simulink model "hf_point_mass_subsonic_airplane"  (R2024b)
settings: Solver=ode45  StartTime=0.0  StopTime=5*60  RelTol=1e-3  AbsTol=1e-6
values from neighbouring files (symbols this model uses):
  FPS2MPH = 3600/5280    (= 0.681818181818)    [luckep2.m]
  RAD2DEG = 180/pi    (= 57.2957795131)    [luckep2.m]
undefined symbols (not defined in the file or in its folder): gd, ic, params
libraries: simulink_extras x5, dspstat3 x1, simulink x1
(part 1 of 2)
settings Model: Creator=jdlarson1  LastModifiedBy=Benjamin Lucke
settings SolverCC: AlgebraicLoopSolver=TrustRegion
settings DataIOCC: SaveFormat=Array  SignalLoggingSaveFormat=ModelDataLogs  ReturnWorkspaceOutputs=off
settings OptimizationCC: BlockReduction=off  BooleanDataType=off  ReuseModelBlockBuffer=off
settings DebuggingCC: SaveWithParameterizedLinksMsg=none  UnderspecifiedInitializationDetection=Classic  MergeDetectMultiDrivingBlocksExec=none  SignalResolutionControl=TryResolveAllWithWarning  MultiTaskDSMMsg=warning  MultiTaskCondExecSysMsg=none  UnconnectedInputMsg=warning  UnconnectedOutputMsg=warning  UnconnectedLineMsg=warning
settings HardwareCC: TargetUnknown=on
settings ModelReferenceCC: EnableRefExpFcnMdlSchedulingChecks=on  PropagateSignalLabelsOutOfModel=off
settings RTWCC: GPUComputeCapability=3.5  DLArmComputeVersion=19.05
settings GRTTargetCC: CombineOutputUpdateFcns=off  GRTInterface=on

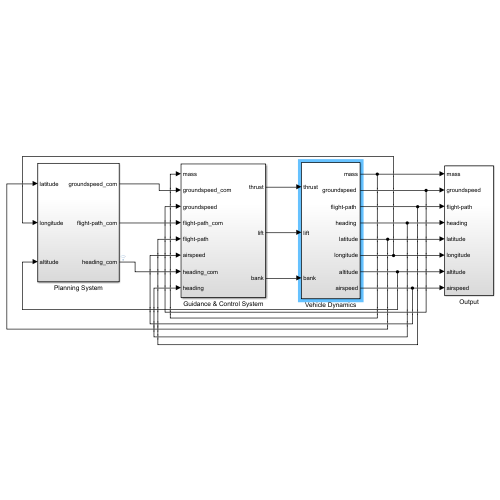
[thumbnail: Simulink's stored preview of the top-level diagram]
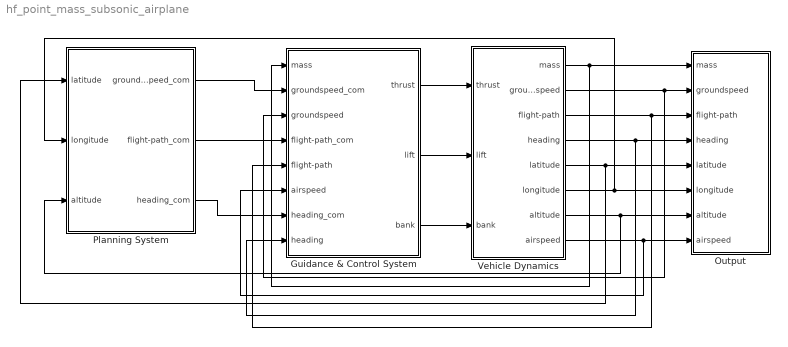
== system hf_point_mass_subsonic_airplane ==
  Guidance & Control System : Subsystem
  Output : Subsystem
  Planning System : Subsystem
  Vehicle Dynamics : Subsystem
  wires:
  Guidance & Control System/3(bank) -> Vehicle Dynamics/3(bank)
  Vehicle Dynamics/1(" mass") -> Output/1(mass), Guidance & Control System/1(mass)
  Guidance & Control System/2(lift) -> Vehicle Dynamics/2("lift ")
  Guidance & Control System/1(thrust) -> Vehicle Dynamics/1("thrust ")
  Planning System/1(groundspeed_com) -> Guidance & Control System/2(groundspeed_com)
  Planning System/2(flight-path_com) -> Guidance & Control System/4(flight-path_com)
  Planning System/3(heading_com) -> Guidance & Control System/7(heading_com)
  Vehicle Dynamics/4(" heading ") -> Guidance & Control System/8(heading), Output/4(heading)
  Vehicle Dynamics/3(" flight-path ") -> Guidance & Control System/5(flight-path), Output/3(flight-path)
  Vehicle Dynamics/2(" groundspeed ") -> Guidance & Control System/3(groundspeed), Output/2(groundspeed)
  Vehicle Dynamics/8(airspeed) -> Guidance & Control System/6(airspeed), Output/8(airspeed)
  Vehicle Dynamics/7(altitude) -> Planning System/3(altitude), Output/7(altitude)
  Vehicle Dynamics/6(longitude) -> Planning System/2(longitude), Output/6(longitude)
  Vehicle Dynamics/5(latitude) -> Planning System/1(latitude), Output/5(latitude)

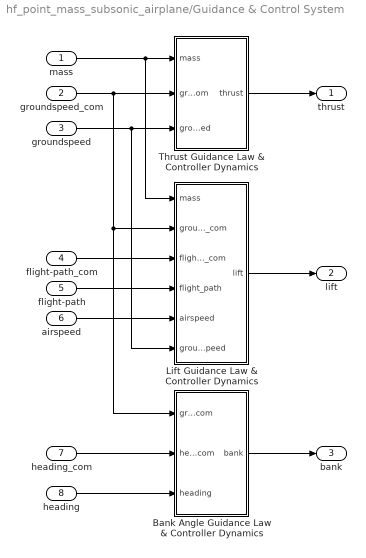
== system hf_point_mass_subsonic_airplane/Guidance & Control System ==
  mass : Inport
  groundspeed_com : Inport  Port=2
  groundspeed : Inport  Port=3
  flight-path_com : Inport  Port=4
  flight-path : Inport  Port=5
  airspeed : Inport  Port=6
  heading_com : Inport  Port=7
  heading : Inport  Port=8
  Bank Angle Guidance Law & Controller Dynamics : Subsystem
  Lift Guidance Law & Controller Dynamics : Subsystem
  Thrust Guidance Law & Controller Dynamics : Subsystem
  thrust : Outport
  lift : Outport  Port=2
  bank : Outport  Port=3
  wires:
  mass/1 -> Lift Guidance Law & Controller Dynamics/1(mass), Thrust Guidance Law & Controller Dynamics/1(mass)
  heading_com/1 -> Bank Angle Guidance Law & Controller Dynamics/2(heading_com)
  groundspeed/1 -> Thrust Guidance Law & Controller Dynamics/3(groundspeed), Lift Guidance Law & Controller Dynamics/6(groundspeed)
  groundspeed_com/1 -> Lift Guidance Law & Controller Dynamics/2(groundspeed_com), Bank Angle Guidance Law & Controller Dynamics/1(groundspeed_com), Thrust Guidance Law & Controller Dynamics/2(groundspeed_com)
  heading/1 -> Bank Angle Guidance Law & Controller Dynamics/3(heading)
  flight-path/1 -> Lift Guidance Law & Controller Dynamics/4(flight_path)
  airspeed/1 -> Lift Guidance Law & Controller Dynamics/5(airspeed)
  Thrust Guidance Law & Controller Dynamics/1(thrust) -> thrust/1
  Lift Guidance Law & Controller Dynamics/1(lift) -> lift/1
  Bank Angle Guidance Law & Controller Dynamics/1(bank) -> bank/1
  flight-path_com/1 -> Lift Guidance Law & Controller Dynamics/3(flight_path_com)

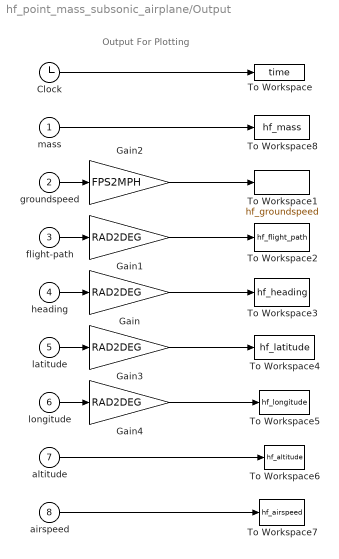
== system hf_point_mass_subsonic_airplane/Output ==
  note: Output For Plotting
  mass : Inport
  groundspeed : Inport  Port=2
  flight-path : Inport  Port=3
  heading : Inport  Port=4
  latitude : Inport  Port=5
  longitude : Inport  Port=6
  altitude : Inport  Port=7
  airspeed : Inport  Port=8
  Clock : Clock
  Gain{,1,3..4} (4 alike) : Gain  Gain=RAD2DEG
  Gain2 : Gain  Gain=FPS2MPH
  To Workspace : ToWorkspace  VariableName=time
  To Workspace1 : ToWorkspace  VariableName=hf_groundspeed
  To Workspace2 : ToWorkspace  VariableName=hf_flight_path
  To Workspace3 : ToWorkspace  VariableName=hf_heading
  To Workspace4 : ToWorkspace  VariableName=hf_latitude
  To Workspace5 : ToWorkspace  VariableName=hf_longitude
  To Workspace6 : ToWorkspace  VariableName=hf_altitude
  To Workspace7 : ToWorkspace  VariableName=hf_airspeed
  To Workspace8 : ToWorkspace  VariableName=hf_mass
  wires:
  Clock/1 -> To Workspace/1
  latitude/1 -> Gain3/1
  groundspeed/1 -> Gain2/1
  flight-path/1 -> Gain1/1
  heading/1 -> Gain/1
  longitude/1 -> Gain4/1
  altitude/1 -> To Workspace6/1
  Gain2/1 -> To Workspace1/1
  Gain1/1 -> To Workspace2/1
  Gain/1 -> To Workspace3/1
  airspeed/1 -> To Workspace7/1
  mass/1 -> To Workspace8/1
  Gain3/1 -> To Workspace4/1
  Gain4/1 -> To Workspace5/1

== system hf_point_mass_subsonic_airplane/Planning System ==
  latitude : Inport
  longitude : Inport  Port=2
  altitude : Inport  Port=3
  CD1 : Gain  Gain=RAD2DEG  SaturateOnIntegerOverflow=on
  CD7 : Gain  Gain=RAD2DEG  SaturateOnIntegerOverflow=on
  CD8 : Gain  Gain=FPS2MPH  SaturateOnIntegerOverflow=on
  Command System : MATLAB Function  TreatAsAtomicUnit=on
  To Workspace10 : ToWorkspace  VariableName=heading_com
  To Workspace5 : ToWorkspace  VariableName=groundspeed_com
  To Workspace7 : ToWorkspace  VariableName=flight_path_com
  groundspeed_com : Outport
  flight-path_com : Outport  Port=2
  heading_com : Outport  Port=3
  wires:
  latitude/1 -> Command System/1(latitude)
  longitude/1 -> Command System/2(longitude)
  altitude/1 -> Command System/3(altitude)
  Command System/1(groundspeed_com) -> CD8/1, groundspeed_com/1
  Command System/2(flight_path_com) -> CD7/1, flight-path_com/1
  Command System/3(heading_com) -> CD1/1, heading_com/1
  CD8/1 -> To Workspace5/1
  CD7/1 -> To Workspace7/1
  CD1/1 -> To Workspace10/1

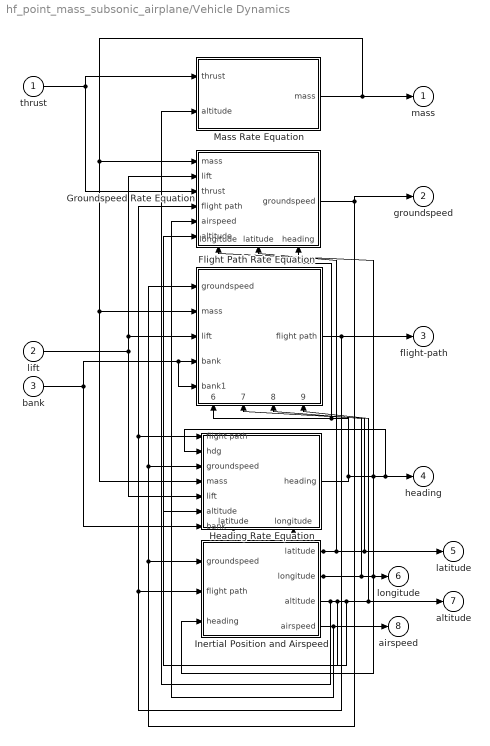
== system hf_point_mass_subsonic_airplane/Vehicle Dynamics ==
  "thrust " : Inport
  "lift " : Inport  Port=2
  bank : Inport  Port=3
  Flight Path Rate Equation : Subsystem
      settings: PortSchema="{\"entries\":[{\"content\":{\"sides\":[{\"content\":{\"connectorIds\":[\"In1\",\"In2\",\"In3\",\"In4\",\"In5\"]},\"type\":\"ConnectorPlacement.EquallySpacedRectSide\",\"uuid\":\"d4397cf0-d6a8-45b4-8ab8-cca84a544394\"},{\"content\":{\"connectorIds\":[\"Out1\"],\"side\":\"RIGHT\"},\"type\":\"ConnectorPlacement.EquallySpacedRectSide\",\"uuid\":\"804857a4-1e47-4b60-94da-14102cd06f3c\"},{\"content\":{\"side\":\"TOP\"},\"type\":\"ConnectorPlacement.EquallySpacedRectSide\",\"uuid\":\"09f0a00a-15e5-437a-b4cb-448802ed4647\"},{\"content\":{\"connectorIds\":[\"In6\",\"In7\",\"In8\",\"In9\"],\"side\":\"BOTTOM\"},\"type\":\"ConnectorPlacement.EquallySpacedRectSide\",\"uuid\":\"1156d38b-a959-4243-b2d5-1a5ac65cda62\"}]},\"type\":\"ConnectorPlacement.EquallySpacedConnector\",\"uuid\":\"d61329f0-9ba5-4e59-b457-f41e73f8c340\"}],\"packageUris\":[\"http://schema.mathworks.com/mf0/Connector/R2020b\"],\"version\":\"1.0\"}"
  Groundspeed Rate Equation : Subsystem
      settings: PortSchema="{\"entries\":[{\"content\":{\"sides\":[{\"content\":{\"connectorIds\":[\"In1\",\"In2\",\"In3\",\"In4\",\"In5\",\"In6\"]},\"type\":\"ConnectorPlacement.EquallySpacedRectSide\",\"uuid\":\"6f7bd2d7-85fc-4563-93ff-9341b9530eba\"},{\"content\":{\"connectorIds\":[\"Out1\"],\"side\":\"RIGHT\"},\"type\":\"ConnectorPlacement.EquallySpacedRectSide\",\"uuid\":\"c7e9f09e-4b99-4546-8d4d-9ca4857fc352\"},{\"content\":{\"side\":\"TOP\"},\"type\":\"ConnectorPlacement.EquallySpacedRectSide\",\"uuid\":\"ec8592c7-5718-4bc6-ac01-24aab67c62ee\"},{\"content\":{\"connectorIds\":[\"In7\",\"In8\",\"In9\"],\"side\":\"BOTTOM\"},\"type\":\"ConnectorPlacement.EquallySpacedRectSide\",\"uuid\":\"788c25ba-363f-4623-ace7-7f08b1fee3bf\"}]},\"type\":\"ConnectorPlacement.EquallySpacedConnector\",\"uuid\":\"7d62769b-4090-428b-8c35-05acd44d5b13\"}],\"packageUris\":[\"http://schema.mathworks.com/mf0/Connector/R2020b\"],\"version\":\"1.0\"}"
  Heading Rate Equation : Subsystem
      settings: PortSchema="{\"entries\":[{\"content\":{\"sides\":[{\"content\":{\"connectorIds\":[\"In1\",\"In2\",\"In3\",\"In4\",\"In5\",\"In6\",\"In7\"]},\"type\":\"ConnectorPlacement.EquallySpacedRectSide\",\"uuid\":\"d596b612-fc07-4863-a50d-995bf54e8f47\"},{\"content\":{\"connectorIds\":[\"Out1\"],\"side\":\"RIGHT\"},\"type\":\"ConnectorPlacement.EquallySpacedRectSide\",\"uuid\":\"c6de21c0-a108-49be-a04c-b12cc2e66be0\"},{\"content\":{\"side\":\"TOP\"},\"type\":\"ConnectorPlacement.EquallySpacedRectSide\",\"uuid\":\"ba0fa9a5-7ccd-45df-afcb-e90b544b3721\"},{\"content\":{\"connectorIds\":[\"In8\",\"In9\"],\"side\":\"BOTTOM\"},\"type\":\"ConnectorPlacement.EquallySpacedRectSide\",\"uuid\":\"6f3d2df9-b18c-4d4a-ac17-7c2083eb4732\"}]},\"type\":\"ConnectorPlacement.EquallySpacedConnector\",\"uuid\":\"41ed9114-5e72-4e94-9929-074f462b6e98\"}],\"packageUris\":[\"http://schema.mathworks.com/mf0/Connector/R2020b\"],\"version\":\"1.0\"}"
  Inertial Position and Airspeed : Subsystem
  Mass Rate Equation : Subsystem
  " mass" : Outport
  " groundspeed " : Outport  Port=2
  " flight-path " : Outport  Port=3
  " heading " : Outport  Port=4
  latitude : Outport  Port=5
  longitude : Outport  Port=6
  altitude : Outport  Port=7
  airspeed : Outport  Port=8
  wires:
  bank/1 -> Heading Rate Equation/7(bank), Flight Path Rate Equation/5(bank1), Flight Path Rate Equation/4(bank)
  "lift "/1 -> Flight Path Rate Equation/3("lift "), Groundspeed Rate Equation/2(lift), Heading Rate Equation/5("lift ")
  "thrust "/1 -> Groundspeed Rate Equation/3(thrust), Mass Rate Equation/1(thrust)
  Heading Rate Equation/1(heading) -> Flight Path Rate Equation/6(heading), Groundspeed Rate Equation/9(heading), Inertial Position and Airspeed/3(heading), Heading Rate Equation/2(hdg), " heading "/1
  Flight Path Rate Equation/1(flight path) -> Groundspeed Rate Equation/4(flight path), Heading Rate Equation/1(flight path), Inertial Position and Airspeed/2("flight path "), " flight-path "/1
  Groundspeed Rate Equation/1(groundspeed) -> " groundspeed "/1, Flight Path Rate Equation/1(groundspeed), Heading Rate Equation/3(groundspeed), Inertial Position and Airspeed/1(groundspeed)
  Inertial Position and Airspeed/2(longitude) -> Groundspeed Rate Equation/7(longitude), longitude/1, Flight Path Rate Equation/8(longitude), Heading Rate Equation/9(longitude)
  Inertial Position and Airspeed/4(airspeed) -> Groundspeed Rate Equation/5(airspeed), airspeed/1
  Inertial Position and Airspeed/1(latitude) -> latitude/1, Flight Path Rate Equation/7(latitude), Groundspeed Rate Equation/8(latitude), Heading Rate Equation/8(latitude)
  Inertial Position and Airspeed/3(altitude) -> Mass Rate Equation/2(altitude), Groundspeed Rate Equation/6(altitude), Heading Rate Equation/6(altitude), Flight Path Rate Equation/9(altitude), altitude/1
  Mass Rate Equation/1("mass ") -> Heading Rate Equation/4(mass), Flight Path Rate Equation/2(mass), Groundspeed Rate Equation/1(mass), " mass"/1

== system hf_point_mass_subsonic_airplane/Guidance & Control System/Bank Angle Guidance Law & Controller Dynamics ==
  groundspeed_com : Inport
  heading_com : Inport  Port=2
  heading : Inport  Port=3
  +- 30 deg saturation : Saturate  UpperLimit=30*pi/180  LowerLimit=-30*pi/180
  Generate roll command : Subsystem
  Inner Loop Bank Dynamics : simulink_extras/Additional Linear/Transfer Fcn (with initial states)  N=[params.wu]  D="[1  params.wu]"  X0=0
  To Workspace : ToWorkspace  VariableName=bank
  To Workspace1 : ToWorkspace  VariableName=bank_com
  bank : Outport
  wires:
  groundspeed_com/1 -> Generate roll command/1(groundspeed_com)
  heading_com/1 -> Generate roll command/2(heading_com)
  heading/1 -> Generate roll command/3(heading)
  Generate roll command/1(mu_command) -> To Workspace1/1, Inner Loop Bank Dynamics/1  "commanded roll"
  Inner Loop Bank Dynamics/1 -> +- 30 deg saturation/1
  +- 30 deg saturation/1 -> bank/1, To Workspace/1  "bank"

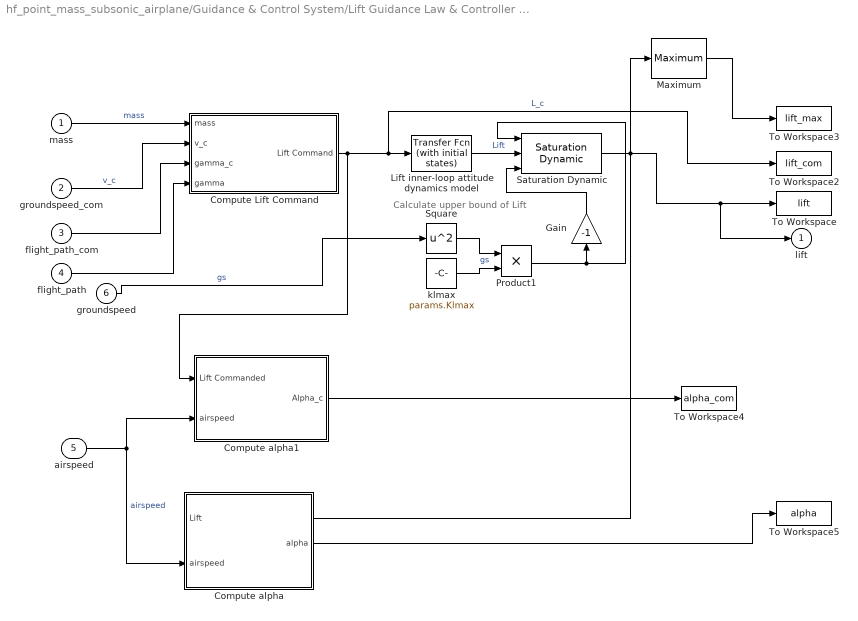
== system hf_point_mass_subsonic_airplane/Guidance & Control System/Lift Guidance Law & Controller Dynamics ==
  note: Calculate upper bound of Lift
  mass : Inport
  groundspeed_com : Inport  Port=2
  flight_path_com : Inport  Port=3
  flight_path : Inport  Port=4
  airspeed : Inport  Port=5
  groundspeed : Inport  Port=6
  Compute Lift Command : Subsystem
  Compute alpha : Subsystem
  Compute alpha1 : Subsystem
  Gain : Gain  Gain=-1
  Lift inner-loop attitude dynamics model : simulink_extras/Additional Linear/Transfer Fcn (with initial states)  N=[params.wl]  D="[1  params.wl]"  X0=0
  Maximum : dspstat3/Maximum  operation=maximum  fcn=Value  indexBase=One  operateOver=Each column  Dimension=1  InputProcessing=Columns as channels (frame based)  reset=None  roiEnable=off  roiType=Rectangles  roiPortion=Entire ROI  roiOutput=Individual statistics for each ROI  roiFlag=off  roundingMode=Floor  overflowMode=off  accumDataTypeStr=Inherit: Same as product output  accumLastDataTypeStr=Inherit: Same as product output
      settings: LibrarySourceBlock=dsphdlsupportstat/Maximum
  Product1 : Product
  Saturation Dynamic : simulink/Discontinuities/Saturation Dynamic  OutMin=[]  OutMax=[]  OutDataTypeStr=Inherit: Same as second input  OutDataType=fixdt(1, 16)  OutScaling=2^-10  DoSatur=off
  Square : Math  Operator=square
  To Workspace : ToWorkspace  VariableName=lift
  To Workspace2 : ToWorkspace  VariableName=lift_com
  To Workspace3 : ToWorkspace  VariableName=lift_max
  To Workspace4 : ToWorkspace  VariableName=alpha_com
  To Workspace5 : ToWorkspace  VariableName=alpha
  klmax : Constant  Value=params.Klmax
  lift : Outport
  wires:
  mass/1 -> Compute Lift Command/1(mass)  "mass"
  groundspeed_com/1 -> Compute Lift Command/2(v_c)  "v_c"
  flight_path_com/1 -> Compute Lift Command/3(gamma_c)
  flight_path/1 -> Compute Lift Command/4(gamma)
  Compute Lift Command/1(Lift Command) -> Compute alpha1/1(Lift Commanded), To Workspace2/1, Lift inner-loop attitude dynamics model/1  "L_c"
  Lift inner-loop attitude dynamics model/1 -> Saturation Dynamic/2  "Lift"
  Maximum/1 -> To Workspace3/1
  groundspeed/1 -> Square/1  "gs"
  Square/1 -> Product1/1  "gs"
  klmax/1 -> Product1/2
  Product1/1 -> Gain/1, Saturation Dynamic/1
  Saturation Dynamic/1 -> Compute alpha/1(Lift), lift/1, To Workspace/1, Maximum/1
  airspeed/1 -> Compute alpha1/2(airspeed), Compute alpha/2(airspeed)  "airspeed"
  Compute alpha1/1(Alpha_c) -> To Workspace4/1
  Compute alpha/1(alpha) -> To Workspace5/1
  Gain/1 -> Saturation Dynamic/3

== system hf_point_mass_subsonic_airplane/Guidance & Control System/Thrust Guidance Law & Controller Dynamics ==
  mass : Inport
  groundspeed_com : Inport  Port=2
  groundspeed : Inport  Port=3
  Generate Thrust Command : Subsystem
  Saturation : Saturate  UpperLimit=params.Tmax  LowerLimit=0
  Thrust inner-loop attitude dynamics model : simulink_extras/Additional Linear/Transfer Fcn (with initial states)  N=[params.wt]  D="[1  params.wt]"  X0=0
  To Workspace : ToWorkspace  VariableName=thrust
  To Workspace1 : ToWorkspace  VariableName=thrust_com
  thrust : Outport
  wires:
  mass/1 -> Generate Thrust Command/1(In1)
  groundspeed_com/1 -> Generate Thrust Command/2(In2)
  groundspeed/1 -> Generate Thrust Command/3(In3)
  Generate Thrust Command/1(Out1) -> To Workspace1/1, Thrust inner-loop attitude dynamics model/1  "thrust_command"
  Thrust inner-loop attitude dynamics model/1 -> Saturation/1  "Thrust"
  Saturation/1 -> thrust/1, To Workspace/1  "Limited Thrust"

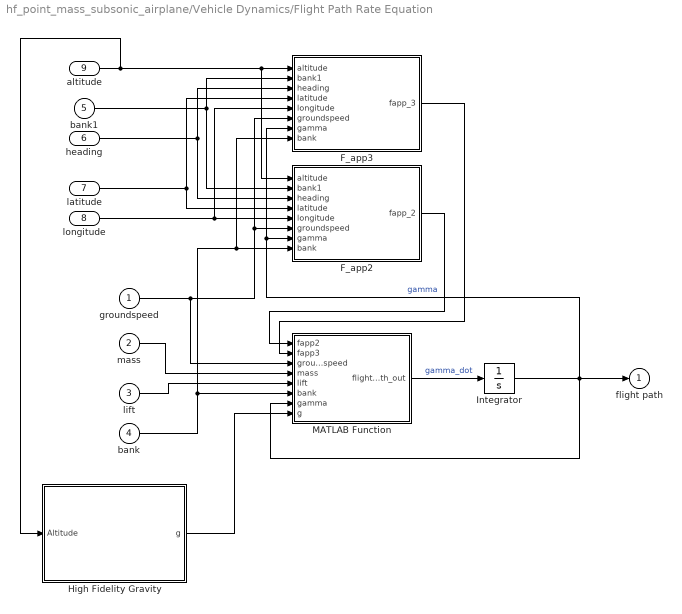
== system hf_point_mass_subsonic_airplane/Vehicle Dynamics/Flight Path Rate Equation ==
  groundspeed : Inport
  mass : Inport  Port=2
  "lift " : Inport  Port=3
  bank : Inport  Port=4
  bank1 : Inport  Port=5
  heading : Inport  Port=6
  latitude : Inport  Port=7
  longitude : Inport  Port=8
  altitude : Inport  Port=9
  F_app2 : Subsystem
  F_app3 : Subsystem
  High Fidelity Gravity : Subsystem
  Integrator : Integrator  InitialCondition=.05
  MATLAB Function : MATLAB Function  TreatAsAtomicUnit=on
  flight path : Outport
  wires:
  groundspeed/1 -> MATLAB Function/3(groundspeed), F_app3/6(groundspeed), F_app2/6(groundspeed)
  mass/1 -> MATLAB Function/4(mass)
  "lift "/1 -> MATLAB Function/5(lift)
  bank/1 -> F_app2/8(bank), F_app3/8(bank), MATLAB Function/6(bank)
  MATLAB Function/1(flight_path_out) -> Integrator/1  "gamma_dot"
  Integrator/1 -> F_app2/7(gamma), F_app3/7(gamma), flight path/1, MATLAB Function/7(gamma)  "gamma"
  altitude/1 -> High Fidelity Gravity/1(Altitude), F_app3/1(altitude), F_app2/1(altitude)
  bank1/1 -> F_app3/2(bank1), F_app2/2(bank1)
  heading/1 -> F_app3/3(heading), F_app2/3(heading)
  latitude/1 -> F_app3/4(latitude), F_app2/4(latitude)
  longitude/1 -> F_app3/5(longitude), F_app2/5(longitude)
  F_app2/1(fapp_2) -> MATLAB Function/1(fapp2)
  F_app3/1(fapp_3) -> MATLAB Function/2(fapp3)
  High Fidelity Gravity/1(g) -> MATLAB Function/8(g)

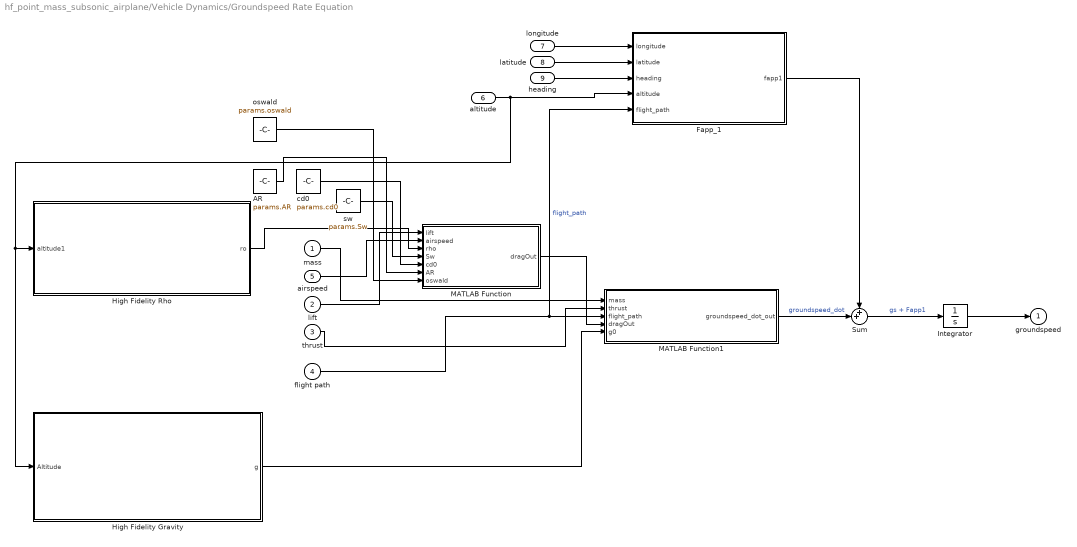
== system hf_point_mass_subsonic_airplane/Vehicle Dynamics/Groundspeed Rate Equation ==
  mass : Inport
  lift : Inport  Port=2
  thrust : Inport  Port=3
  flight path : Inport  Port=4
  airspeed : Inport  Port=5
  altitude : Inport  Port=6
  longitude : Inport  Port=7
  latitude : Inport  Port=8
  heading : Inport  Port=9
  AR : Constant  Value=params.AR
  Fapp_1 : Subsystem
  High Fidelity Gravity : Subsystem
  High Fidelity Rho : Subsystem
  Integrator : Integrator  InitialCondition=600
  MATLAB Function : MATLAB Function  TreatAsAtomicUnit=on
  MATLAB Function1 : MATLAB Function  TreatAsAtomicUnit=on
  Sum : Sum  Inputs=++|
  cd0 : Constant  Value=params.cd0
  oswald : Constant  Value=params.oswald
  sw : Constant  Value=params.Sw
  groundspeed : Outport
  wires:
  lift/1 -> MATLAB Function/1(lift)
  airspeed/1 -> MATLAB Function/2(airspeed)
  mass/1 -> MATLAB Function1/1(mass)
  thrust/1 -> MATLAB Function1/2(thrust)
  flight path/1 -> Fapp_1/5(flight_path), MATLAB Function1/3(flight_path)  "flight_path"
  MATLAB Function/1(dragOut) -> MATLAB Function1/4(dragOut)
  sw/1 -> MATLAB Function/4(Sw)
  cd0/1 -> MATLAB Function/5(cd0)
  AR/1 -> MATLAB Function/6(AR)
  oswald/1 -> MATLAB Function/7(oswald)
  longitude/1 -> Fapp_1/1(longitude)
  latitude/1 -> Fapp_1/2(latitude)
  heading/1 -> Fapp_1/3(heading)
  altitude/1 -> High Fidelity Gravity/1(Altitude), High Fidelity Rho/1(altitude1), Fapp_1/4(altitude)
  High Fidelity Rho/1(ro) -> MATLAB Function/3(rho)
  MATLAB Function1/1(groundspeed_dot_out) -> Sum/2  "groundspeed_dot"
  Fapp_1/1(fapp1) -> Sum/1
  Sum/1 -> Integrator/1  "gs + Fapp1"
  High Fidelity Gravity/1(g) -> MATLAB Function1/5(g0)
  Integrator/1 -> groundspeed/1

== system hf_point_mass_subsonic_airplane/Vehicle Dynamics/Heading Rate Equation ==
  flight path : Inport
  hdg : Inport  Port=2
  groundspeed : Inport  Port=3
  mass : Inport  Port=4
  "lift " : Inport  Port=5
  altitude : Inport  Port=6
  bank : Inport  Port=7
  latitude : Inport  Port=8
  longitude : Inport  Port=9
  F_app2 : Subsystem
  F_app3 : Subsystem
  Integrator : Integrator  InitialCondition=.003
  MATLAB Function : MATLAB Function  TreatAsAtomicUnit=on
  heading : Outport
  wires:
  altitude/1 -> F_app2/1(altitude), F_app3/1(altitude)
  hdg/1 -> F_app3/2(heading), F_app2/2(heading)
  latitude/1 -> F_app3/3(latitude), F_app2/3(latitude)
  longitude/1 -> F_app2/4(longitude), F_app3/4(longitude)
  mass/1 -> MATLAB Function/5(mass)
  bank/1 -> F_app2/7(bank), MATLAB Function/7(bank), F_app3/7(bank)
  flight path/1 -> MATLAB Function/3(flight_path), F_app2/6(gamma), F_app3/6(gamma)
  groundspeed/1 -> MATLAB Function/4(groundspeed), F_app2/5(groundspeed), F_app3/5(groundspeed)
  "lift "/1 -> MATLAB Function/6(lift)
  MATLAB Function/1(heading_out) -> Integrator/1  "sigma-dot"
  Integrator/1 -> heading/1  "sigma"
  F_app2/1(fapp_2) -> MATLAB Function/1(fapp2)
  F_app3/1(fapp_3) -> MATLAB Function/2(fapp3)

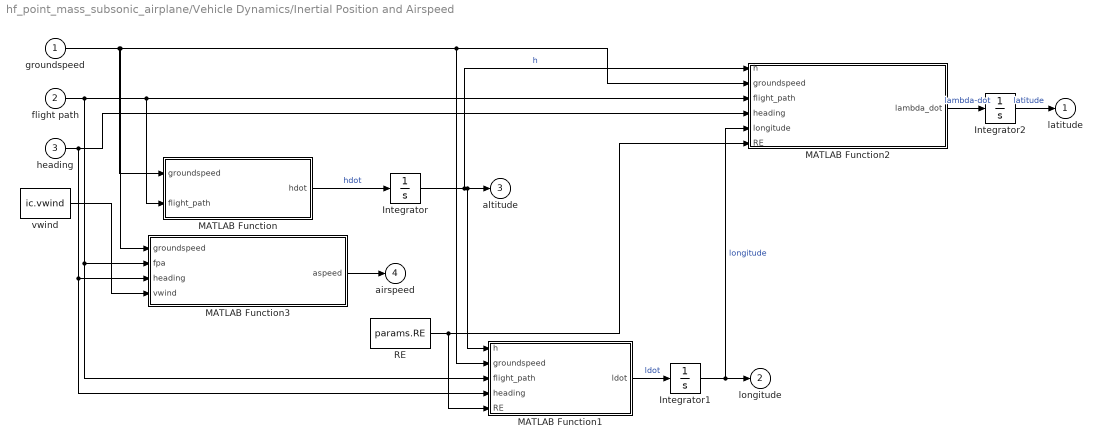
== system hf_point_mass_subsonic_airplane/Vehicle Dynamics/Inertial Position and Airspeed ==
  groundspeed : Inport
  "flight path " : Inport  Port=2
  heading : Inport  Port=3
  Integrator : Integrator  InitialCondition=20000
  Integrator1 : Integrator  InitialCondition=33.2098
  Integrator2 : Integrator  InitialCondition=-87.5692
  MATLAB Function : MATLAB Function  TreatAsAtomicUnit=on
  MATLAB Function1 : MATLAB Function  TreatAsAtomicUnit=on
  MATLAB Function2 : MATLAB Function  TreatAsAtomicUnit=on
  MATLAB Function3 : MATLAB Function  TreatAsAtomicUnit=on
  RE : Constant  Value=params.RE
  vwind : Constant  Value=ic.vwind
  latitude : Outport
  longitude : Outport  Port=2
  altitude : Outport  Port=3
  airspeed : Outport  Port=4
  wires:
  heading/1 -> MATLAB Function3/3(heading), MATLAB Function1/4(heading), MATLAB Function2/4(heading)
  Integrator1/1 -> longitude/1, MATLAB Function2/5(longitude)  "longitude"
  "flight path "/1 -> MATLAB Function1/3(flight_path), MATLAB Function3/2(fpa), MATLAB Function2/3(flight_path), MATLAB Function/2(flight_path)
  groundspeed/1 -> MATLAB Function1/2(groundspeed), MATLAB Function2/2(groundspeed), MATLAB Function3/1(groundspeed), MATLAB Function/1(groundspeed)
  RE/1 -> MATLAB Function2/6(RE), MATLAB Function1/5(RE)
  vwind/1 -> MATLAB Function3/4(vwind)
  Integrator/1 -> MATLAB Function1/1(h), altitude/1, MATLAB Function2/1(h)  "h"
  MATLAB Function/1(hdot) -> Integrator/1  "hdot"
  MATLAB Function3/1(aspeed) -> airspeed/1
  MATLAB Function1/1(ldot) -> Integrator1/1  "ldot"
  MATLAB Function2/1(lambda_dot) -> Integrator2/1  "lambda-dot"
  Integrator2/1 -> latitude/1  "latitude"

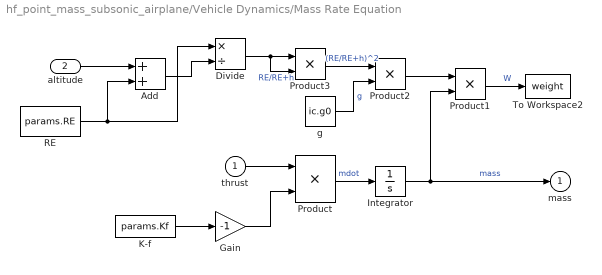
== system hf_point_mass_subsonic_airplane/Vehicle Dynamics/Mass Rate Equation ==
  thrust : Inport
  altitude : Inport  Port=2
  Add : Sum
  Divide : Product  Inputs=*/
  Gain : Gain  Gain=-1
  Integrator : Integrator  InitialCondition=200000
  K-f : Constant  Value=params.Kf
  Product{,1..3} (4 alike) : Product
  RE : Constant  Value=params.RE
  To Workspace2 : ToWorkspace  VariableName=weight
  g : Constant  Value=ic.g0
  "mass " : Outport
  wires:
  Divide/1 -> Product3/2, Product3/1  "RE/RE+h"
  RE/1 -> Divide/1, Add/2
  Add/1 -> Divide/2
  Product1/1 -> To Workspace2/1  "W"
  altitude/1 -> Add/1
  thrust/1 -> Product/1
  K-f/1 -> Gain/1
  Gain/1 -> Product/2
  Product3/1 -> Product2/1  "(RE/RE+h)^2"
  g/1 -> Product2/2  "g"
  Product/1 -> Integrator/1  "mdot"
  Product2/1 -> Product1/1
  Integrator/1 -> Product1/2, "mass "/1  "mass"

== system hf_point_mass_subsonic_airplane/Guidance & Control System/Bank Angle Guidance Law & Controller Dynamics/Generate roll command ==
  groundspeed_com : Inport
  heading_com : Inport  Port=2
  heading : Inport  Port=3
  Divide : Product  Inputs=*/
  K_up : Gain  Gain=gd.Kup
  Mass1 : Constant  Value=ic.g0
  Product : Product
  Subtract : Sum  Inputs=+-
  mu_command : Outport
  wires:
  groundspeed_com/1 -> Divide/1
  Mass1/1 -> Divide/2
  Subtract/1 -> Product/2  "sigma_c - sigma"
  heading_com/1 -> Subtract/1
  heading/1 -> Subtract/2
  Divide/1 -> K_up/1
  K_up/1 -> Product/1
  Product/1 -> mu_command/1  "mu_command"

== system hf_point_mass_subsonic_airplane/Guidance & Control System/Lift Guidance Law & Controller Dynamics/Compute Lift Command ==
  mass : Inport
  v_c : Inport  Port=2
  gamma_c : Inport  Port=3
  gamma : Inport  Port=4
  PI Thrust Controller : simulink_extras/Additional Linear/Transfer Fcn (with initial states)  N=[gd.Klp gd.Kli]  D="[1  0]"  X0=0
  Product : Product  Inputs=3
  compute sin difference : MATLAB Function  TreatAsAtomicUnit=on
  Lift Command : Outport
  wires:
  compute sin difference/1(y) -> Product/3
  Product/1 -> PI Thrust Controller/1
  gamma/1 -> compute sin difference/2(gamma)
  mass/1 -> Product/1
  v_c/1 -> Product/2
  gamma_c/1 -> compute sin difference/1(gamma_c)
  PI Thrust Controller/1 -> Lift Command/1  "Lift command"

== system hf_point_mass_subsonic_airplane/Guidance & Control System/Lift Guidance Law & Controller Dynamics/Compute alpha ==
  Lift : Inport
  airspeed : Inport  Port=2
  2/rho/sw/cla : MATLAB Function  TreatAsAtomicUnit=on
  Add : Sum
  Density : Constant  Value=ic.rho
  Divide : Product  Inputs=*/
  Product : Product
  Wing load : Constant  Value=params.Sw
  alpha_0 : Constant  Value=params.a0
  lift slope : Constant  Value=params.cla
  alpha : Outport
  wires:
  Add/1 -> alpha/1  "alpha"
  2/rho/sw/cla/1(y) -> Product/2
  Density/1 -> 2/rho/sw/cla/1(rho)
  airspeed/1 -> Divide/2
  Lift/1 -> Divide/1
  Divide/1 -> Product/1
  lift slope/1 -> 2/rho/sw/cla/3(cla)
  Wing load/1 -> 2/rho/sw/cla/2(sw)
  Product/1 -> Add/1
  alpha_0/1 -> Add/2

== system hf_point_mass_subsonic_airplane/Guidance & Control System/Lift Guidance Law & Controller Dynamics/Compute alpha1 ==
  Lift Commanded : Inport
  airspeed : Inport  Port=2
  2/rho/sw/cla : MATLAB Function  TreatAsAtomicUnit=on
  Add : Sum
  Density : Constant  Value=ic.rho
  Divide : Product  Inputs=*/
  Product : Product
  Wing load : Constant  Value=params.Sw
  alpha_0 : Constant  Value=params.a0
  lift slope : Constant  Value=params.cla
  Alpha_c : Outport
  wires:
  alpha_0/1 -> Add/2
  Product/1 -> Add/1
  Wing load/1 -> 2/rho/sw/cla/2(sw)
  lift slope/1 -> 2/rho/sw/cla/3(cla)
  Divide/1 -> Product/1
  Lift Commanded/1 -> Divide/1
  airspeed/1 -> Divide/2
  Density/1 -> 2/rho/sw/cla/1(rho)
  2/rho/sw/cla/1(y) -> Product/2
  Add/1 -> Alpha_c/1  "alpha"

== system hf_point_mass_subsonic_airplane/Guidance & Control System/Thrust Guidance Law & Controller Dynamics/Generate Thrust Command ==
  In1 : Inport
  In2 : Inport  Port=2
  In3 : Inport  Port=3
  Add : Sum  Inputs=+-
  PI Thrust Controller : simulink_extras/Additional Linear/Transfer Fcn (with initial states)  N=[gd.Ktp gd.Kti]  D="[1  0]"  X0=0
  Product : Product
  Out1 : Outport
  wires:
  Product/1 -> PI Thrust Controller/1
  Add/1 -> Product/2
  PI Thrust Controller/1 -> Out1/1  "Thrust command"
  In3/1 -> Add/2  "Groundspeed actual"
  In1/1 -> Product/1  "Mass"
  In2/1 -> Add/1  "Groundspeed Command"

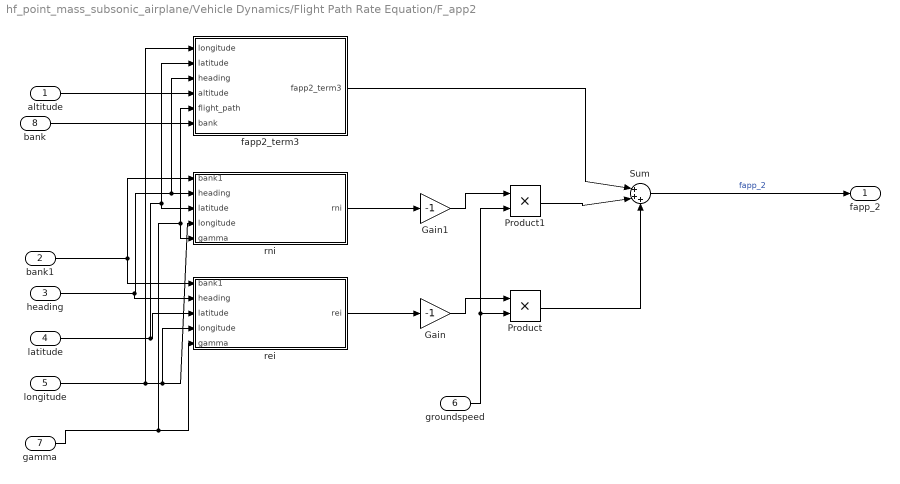
== system hf_point_mass_subsonic_airplane/Vehicle Dynamics/Flight Path Rate Equation/F_app2 ==
  altitude : Inport
  bank1 : Inport  Port=2
  heading : Inport  Port=3
  latitude : Inport  Port=4
  longitude : Inport  Port=5
  groundspeed : Inport  Port=6
  gamma : Inport  Port=7
  bank : Inport  Port=8
  Gain : Gain  Gain=-1
  Gain1 : Gain  Gain=-1
  Product : Product
  Product1 : Product
  Sum : Sum  Inputs=|+++
  fapp2_term3 : Subsystem
  rei : Subsystem
  rni : Subsystem
  fapp_2 : Outport
  wires:
  gamma/1 -> rei/5(gamma), fapp2_term3/5(flight_path), rni/5(gamma)
  latitude/1 -> rei/3(latitude), fapp2_term3/2(latitude), rni/3(latitude)
  Product/1 -> Sum/3
  heading/1 -> rei/2(heading), fapp2_term3/3(heading), rni/2(heading)
  fapp2_term3/1(fapp2_term3) -> Sum/1
  Gain/1 -> Product/1
  bank1/1 -> rei/1(bank1), rni/1(bank1)
  longitude/1 -> fapp2_term3/1(longitude), rei/4(longitude), rni/4(longitude)
  Gain1/1 -> Product1/1
  rni/1(rni) -> Gain1/1
  groundspeed/1 -> Product1/2, Product/2
  rei/1(rei) -> Gain/1
  Sum/1 -> fapp_2/1  "fapp_2"
  Product1/1 -> Sum/2
  altitude/1 -> fapp2_term3/4(altitude)
  bank/1 -> fapp2_term3/6(bank)

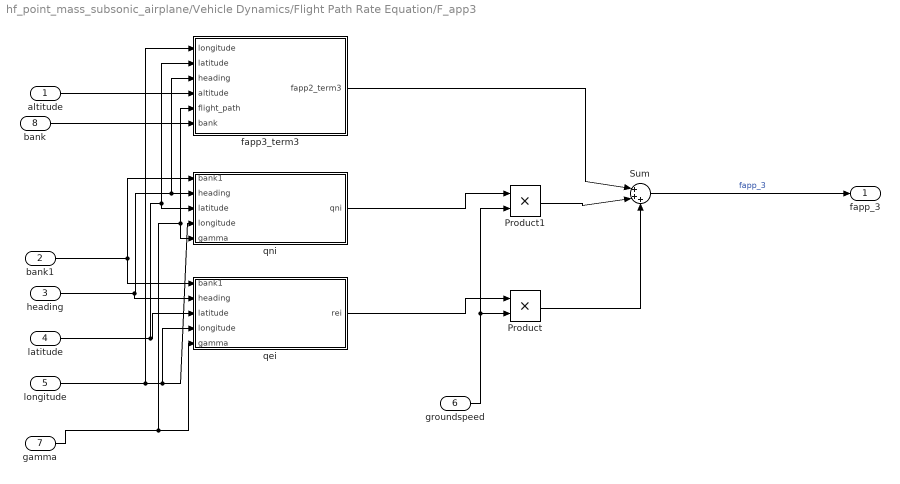
== system hf_point_mass_subsonic_airplane/Vehicle Dynamics/Flight Path Rate Equation/F_app3 ==
  altitude : Inport
  bank1 : Inport  Port=2
  heading : Inport  Port=3
  latitude : Inport  Port=4
  longitude : Inport  Port=5
  groundspeed : Inport  Port=6
  gamma : Inport  Port=7
  bank : Inport  Port=8
  Product : Product
  Product1 : Product
  Sum : Sum  Inputs=|+++
  fapp3_term3 : Subsystem
  qei : Subsystem
  qni : Subsystem
  fapp_3 : Outport
  wires:
  gamma/1 -> qei/5(gamma), fapp3_term3/5(flight_path), qni/5(gamma)
  latitude/1 -> qei/3(latitude), fapp3_term3/2(latitude), qni/3(latitude)
  Product/1 -> Sum/3
  heading/1 -> qei/2(heading), fapp3_term3/3(heading), qni/2(heading)
  fapp3_term3/1(fapp2_term3) -> Sum/1
  qei/1(rei) -> Product/1
  bank1/1 -> qei/1(bank1), qni/1(bank1)
  longitude/1 -> fapp3_term3/1(longitude), qei/4(longitude), qni/4(longitude)
  qni/1(qni) -> Product1/1
  groundspeed/1 -> Product1/2, Product/2
  Sum/1 -> fapp_3/1  "fapp_3"
  Product1/1 -> Sum/2
  altitude/1 -> fapp3_term3/4(altitude)
  bank/1 -> fapp3_term3/6(bank)

== system hf_point_mass_subsonic_airplane/Vehicle Dynamics/Flight Path Rate Equation/High Fidelity Gravity ==
  Altitude : Inport
  Add : Sum
  Constant1 : Constant  Value=ic.g0
  Divide : Product  Inputs=*/
  Product2 : Product
  Product3 : Product
  RE : Constant  Value=params.RE
  g : Outport
  wires:
  Add/1 -> Divide/2
  Constant1/1 -> Product2/2
  Divide/1 -> Product3/1, Product3/2  "RE/RE+h"
  Product3/1 -> Product2/1  "(RE/RE+h)^2"
  Product2/1 -> g/1  "go re/re+h ^2"
  RE/1 -> Divide/1, Add/1
  Altitude/1 -> Add/2

== system hf_point_mass_subsonic_airplane/Vehicle Dynamics/Groundspeed Rate Equation/Fapp_1 ==
  longitude : Inport
  latitude : Inport  Port=2
  heading : Inport  Port=3
  altitude : Inport  Port=4
  flight_path : Inport  Port=5
  MATLAB Function2 : MATLAB Function  TreatAsAtomicUnit=on
  RE : Constant  Value=params.RE
  w_earth : Constant  Value=7.2921159e-5
  fapp1 : Outport
  wires:
  heading/1 -> MATLAB Function2/3(heading)
  w_earth/1 -> MATLAB Function2/4(w_e)
  altitude/1 -> MATLAB Function2/5(altitude)
  MATLAB Function2/1(fapp1) -> fapp1/1
  latitude/1 -> MATLAB Function2/2(latitude)
  longitude/1 -> MATLAB Function2/1(longitude)
  RE/1 -> MATLAB Function2/6(RE)
  flight_path/1 -> MATLAB Function2/7(flight_path)

== system hf_point_mass_subsonic_airplane/Vehicle Dynamics/Groundspeed Rate Equation/High Fidelity Gravity ==
  Altitude : Inport
  Add : Sum
  Constant1 : Constant  Value=ic.g0
  Divide : Product  Inputs=*/
  Product2 : Product
  Product3 : Product
  RE : Constant  Value=params.RE
  g : Outport
  wires:
  Add/1 -> Divide/2
  Constant1/1 -> Product2/2
  Divide/1 -> Product3/1, Product3/2  "RE/RE+h"
  RE/1 -> Divide/1, Add/2
  Product3/1 -> Product2/1  "(RE/RE+h)^2"
  Product2/1 -> g/1  "go re/re+h ^2"
  Altitude/1 -> Add/1

== system hf_point_mass_subsonic_airplane/Vehicle Dynamics/Groundspeed Rate Equation/High Fidelity Rho ==
  altitude1 : Inport
  MATLAB Function2 : MATLAB Function  TreatAsAtomicUnit=on
  ro : Outport
  wires:
  altitude1/1 -> MATLAB Function2/1(altitude)
  MATLAB Function2/1(ro) -> ro/1

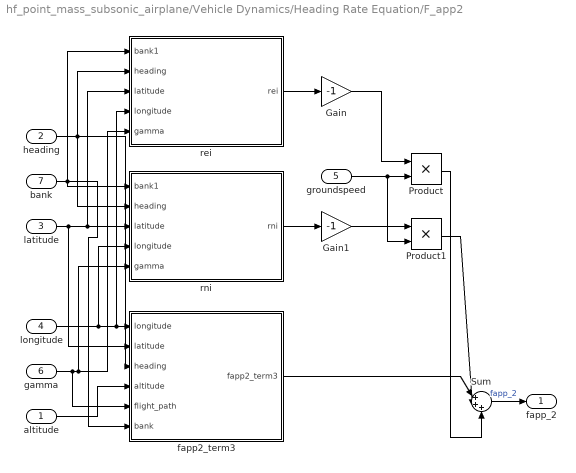
== system hf_point_mass_subsonic_airplane/Vehicle Dynamics/Heading Rate Equation/F_app2 ==
  altitude : Inport
  heading : Inport  Port=2
  latitude : Inport  Port=3
  longitude : Inport  Port=4
  groundspeed : Inport  Port=5
  gamma : Inport  Port=6
  bank : Inport  Port=7
  Gain : Gain  Gain=-1
  Gain1 : Gain  Gain=-1
  Product : Product
  Product1 : Product
  Sum : Sum  Inputs=|+++
  fapp2_term3 : Subsystem
  rei : Subsystem
  rni : Subsystem
  fapp_2 : Outport
  wires:
  rei/1(rei) -> Gain/1
  longitude/1 -> rei/4(longitude), fapp2_term3/1(longitude), rni/4(longitude)
  altitude/1 -> fapp2_term3/4(altitude)
  gamma/1 -> rni/5(gamma), rei/5(gamma), fapp2_term3/5(flight_path)
  Product1/1 -> Sum/2
  heading/1 -> fapp2_term3/3(heading), rni/2(heading), rei/2(heading)
  latitude/1 -> rni/3(latitude), rei/3(latitude), fapp2_term3/2(latitude)
  bank/1 -> fapp2_term3/6(bank), rni/1(bank1), rei/1(bank1)
  rni/1(rni) -> Gain1/1
  fapp2_term3/1(fapp2_term3) -> Sum/1
  Sum/1 -> fapp_2/1  "fapp_2"
  Gain/1 -> Product/1
  groundspeed/1 -> Product1/2, Product/2
  Gain1/1 -> Product1/1
  Product/1 -> Sum/3

== system hf_point_mass_subsonic_airplane/Vehicle Dynamics/Heading Rate Equation/F_app3 ==
  altitude : Inport
  heading : Inport  Port=2
  latitude : Inport  Port=3
  longitude : Inport  Port=4
  groundspeed : Inport  Port=5
  gamma : Inport  Port=6
  bank : Inport  Port=7
  Product : Product
  Product1 : Product
  Sum : Sum  Inputs=|+++
  fapp3_term3 : Subsystem
  qei : Subsystem
  qni : Subsystem
  fapp_3 : Outport
  wires:
  fapp3_term3/1(fapp2_term3) -> Sum/1
  gamma/1 -> qni/5(gamma), qei/5(gamma), fapp3_term3/5(flight_path)
  longitude/1 -> qni/4(longitude), fapp3_term3/1(longitude), qei/4(longitude)
  heading/1 -> fapp3_term3/3(heading), qni/2(heading), qei/2(heading)
  latitude/1 -> qni/3(latitude), qei/3(latitude), fapp3_term3/2(latitude)
  bank/1 -> fapp3_term3/6(bank), qei/1(bank1), qni/1(bank1)
  qei/1(rei) -> Product/1
  altitude/1 -> fapp3_term3/4(altitude)
  qni/1(qni) -> Product1/1
  groundspeed/1 -> Product1/2, Product/2
  Product1/1 -> Sum/2
  Product/1 -> Sum/3
  Sum/1 -> fapp_3/1  "fapp_3"

== system hf_point_mass_subsonic_airplane/Vehicle Dynamics/Flight Path Rate Equation/F_app2/fapp2_term3 ==
  longitude : Inport
  latitude : Inport  Port=2
  heading : Inport  Port=3
  altitude : Inport  Port=4
  flight_path : Inport  Port=5
  bank : Inport  Port=6
  MATLAB Function2 : MATLAB Function  TreatAsAtomicUnit=on
  RE : Constant  Value=params.RE
  w_earth : Constant  Value=7.2921159e-5
  fapp2_term3 : Outport
  wires:
  heading/1 -> MATLAB Function2/3(heading)
  w_earth/1 -> MATLAB Function2/4(w_e)
  altitude/1 -> MATLAB Function2/5(altitude)
  MATLAB Function2/1(fapp2) -> fapp2_term3/1
  latitude/1 -> MATLAB Function2/2(latitude)
  longitude/1 -> MATLAB Function2/1(longitude)
  RE/1 -> MATLAB Function2/6(RE)
  flight_path/1 -> MATLAB Function2/8(flight_path)
  bank/1 -> MATLAB Function2/7(bank)

== system hf_point_mass_subsonic_airplane/Vehicle Dynamics/Flight Path Rate Equation/F_app2/rei ==
  bank1 : Inport
  heading : Inport  Port=2
  latitude : Inport  Port=3
  longitude : Inport  Port=4
  gamma : Inport  Port=5
  get rei : MATLAB Function  TreatAsAtomicUnit=on
  w_earth : Constant  Value=7.2921159e-5
  rei : Outport
  wires:
  w_earth/1 -> get rei/4(we)
  longitude/1 -> get rei/6(longitude)
  bank1/1 -> get rei/1(bank)
  heading/1 -> get rei/3(heading)
  gamma/1 -> get rei/2(fpa)
  latitude/1 -> get rei/5(latitude)
  get rei/1(rei) -> rei/1

== system hf_point_mass_subsonic_airplane/Vehicle Dynamics/Flight Path Rate Equation/F_app2/rni ==
  bank1 : Inport
  heading : Inport  Port=2
  latitude : Inport  Port=3
  longitude : Inport  Port=4
  gamma : Inport  Port=5
  get r_ni : MATLAB Function  TreatAsAtomicUnit=on
  w_earth : Constant  Value=7.2921159e-5
  rni : Outport
  wires:
  get r_ni/1(rni) -> rni/1
  latitude/1 -> get r_ni/5(latitude)
  gamma/1 -> get r_ni/2(fpa)
  heading/1 -> get r_ni/3(heading)
  bank1/1 -> get r_ni/1(bank)
  longitude/1 -> get r_ni/6(longitude)
  w_earth/1 -> get r_ni/4(we)

== system hf_point_mass_subsonic_airplane/Vehicle Dynamics/Flight Path Rate Equation/F_app3/fapp3_term3 ==
  longitude : Inport
  latitude : Inport  Port=2
  heading : Inport  Port=3
  altitude : Inport  Port=4
  flight_path : Inport  Port=5
  bank : Inport  Port=6
  MATLAB Function2 : MATLAB Function  TreatAsAtomicUnit=on
  RE : Constant  Value=params.RE
  w_earth : Constant  Value=7.2921159e-5
  fapp2_term3 : Outport
  wires:
  heading/1 -> MATLAB Function2/3(heading)
  w_earth/1 -> MATLAB Function2/4(w_e)
  altitude/1 -> MATLAB Function2/5(altitude)
  MATLAB Function2/1(fapp3) -> fapp2_term3/1
  latitude/1 -> MATLAB Function2/2(latitude)
  longitude/1 -> MATLAB Function2/1(longitude)
  RE/1 -> MATLAB Function2/6(RE)
  flight_path/1 -> MATLAB Function2/8(flight_path)
  bank/1 -> MATLAB Function2/7(bank)

== system hf_point_mass_subsonic_airplane/Vehicle Dynamics/Flight Path Rate Equation/F_app3/qei ==
  bank1 : Inport
  heading : Inport  Port=2
  latitude : Inport  Port=3
  longitude : Inport  Port=4
  gamma : Inport  Port=5
  get qei : MATLAB Function  TreatAsAtomicUnit=on
  w_earth : Constant  Value=7.2921159e-5
  rei : Outport
  wires:
  w_earth/1 -> get qei/4(we)
  longitude/1 -> get qei/6(longitude)
  bank1/1 -> get qei/1(bank)
  heading/1 -> get qei/3(heading)
  gamma/1 -> get qei/2(fpa)
  latitude/1 -> get qei/5(latitude)
  get qei/1(qei) -> rei/1

== system hf_point_mass_subsonic_airplane/Vehicle Dynamics/Flight Path Rate Equation/F_app3/qni ==
  bank1 : Inport
  heading : Inport  Port=2
  latitude : Inport  Port=3
  longitude : Inport  Port=4
  gamma : Inport  Port=5
  get qni : MATLAB Function  TreatAsAtomicUnit=on
  w_earth : Constant  Value=7.2921159e-5
  qni : Outport
  wires:
  get qni/1(qni) -> qni/1
  latitude/1 -> get qni/5(latitude)
  gamma/1 -> get qni/2(fpa)
  heading/1 -> get qni/3(heading)
  bank1/1 -> get qni/1(bank)
  longitude/1 -> get qni/6(longitude)
  w_earth/1 -> get qni/4(we)

== system hf_point_mass_subsonic_airplane/Vehicle Dynamics/Heading Rate Equation/F_app2/fapp2_term3 ==
  longitude : Inport
  latitude : Inport  Port=2
  heading : Inport  Port=3
  altitude : Inport  Port=4
  flight_path : Inport  Port=5
  bank : Inport  Port=6
  MATLAB Function2 : MATLAB Function  TreatAsAtomicUnit=on
  RE : Constant  Value=params.RE
  w_earth : Constant  Value=7.2921159e-5
  fapp2_term3 : Outport
  wires:
  longitude/1 -> MATLAB Function2/1(longitude)
  latitude/1 -> MATLAB Function2/2(latitude)
  flight_path/1 -> MATLAB Function2/8(flight_path)
  heading/1 -> MATLAB Function2/3(heading)
  w_earth/1 -> MATLAB Function2/4(w_e)
  bank/1 -> MATLAB Function2/7(bank)
  MATLAB Function2/1(fapp2) -> fapp2_term3/1
  altitude/1 -> MATLAB Function2/5(altitude)
  RE/1 -> MATLAB Function2/6(RE)

== system hf_point_mass_subsonic_airplane/Vehicle Dynamics/Heading Rate Equation/F_app2/rei ==
  bank1 : Inport
  heading : Inport  Port=2
  latitude : Inport  Port=3
  longitude : Inport  Port=4
  gamma : Inport  Port=5
  get rei : MATLAB Function  TreatAsAtomicUnit=on
  w_earth : Constant  Value=7.2921159e-5
  rei : Outport
  wires:
  bank1/1 -> get rei/1(bank)
  latitude/1 -> get rei/5(latitude)
  gamma/1 -> get rei/2(fpa)
  longitude/1 -> get rei/6(longitude)
  heading/1 -> get rei/3(heading)
  w_earth/1 -> get rei/4(we)
  get rei/1(rei) -> rei/1

== system hf_point_mass_subsonic_airplane/Vehicle Dynamics/Heading Rate Equation/F_app2/rni ==
  bank1 : Inport
  heading : Inport  Port=2
  latitude : Inport  Port=3
  longitude : Inport  Port=4
  gamma : Inport  Port=5
  get r_ni : MATLAB Function  TreatAsAtomicUnit=on
  w_earth : Constant  Value=7.2921159e-5
  rni : Outport
  wires:
  w_earth/1 -> get r_ni/4(we)
  bank1/1 -> get r_ni/1(bank)
  get r_ni/1(rni) -> rni/1
  latitude/1 -> get r_ni/5(latitude)
  gamma/1 -> get r_ni/2(fpa)
  longitude/1 -> get r_ni/6(longitude)
  heading/1 -> get r_ni/3(heading)

== system hf_point_mass_subsonic_airplane/Vehicle Dynamics/Heading Rate Equation/F_app3/fapp3_term3 ==
  longitude : Inport
  latitude : Inport  Port=2
  heading : Inport  Port=3
  altitude : Inport  Port=4
  flight_path : Inport  Port=5
  bank : Inport  Port=6
  MATLAB Function2 : MATLAB Function  TreatAsAtomicUnit=on
  RE : Constant  Value=params.RE
  w_earth : Constant  Value=7.2921159e-5
  fapp2_term3 : Outport
  wires:
  bank/1 -> MATLAB Function2/7(bank)
  altitude/1 -> MATLAB Function2/5(altitude)
  latitude/1 -> MATLAB Function2/2(latitude)
  longitude/1 -> MATLAB Function2/1(longitude)
  flight_path/1 -> MATLAB Function2/8(flight_path)
  heading/1 -> MATLAB Function2/3(heading)
  w_earth/1 -> MATLAB Function2/4(w_e)
  RE/1 -> MATLAB Function2/6(RE)
  MATLAB Function2/1(fapp3) -> fapp2_term3/1

== system hf_point_mass_subsonic_airplane/Vehicle Dynamics/Heading Rate Equation/F_app3/qei ==
  bank1 : Inport
  heading : Inport  Port=2
  latitude : Inport  Port=3
  longitude : Inport  Port=4
  gamma : Inport  Port=5
  get qei : MATLAB Function  TreatAsAtomicUnit=on
  w_earth : Constant  Value=7.2921159e-5
  rei : Outport
  wires:
  w_earth/1 -> get qei/4(we)
  bank1/1 -> get qei/1(bank)
  get qei/1(qei) -> rei/1
  latitude/1 -> get qei/5(latitude)
  gamma/1 -> get qei/2(fpa)
  longitude/1 -> get qei/6(longitude)
  heading/1 -> get qei/3(heading)

== system hf_point_mass_subsonic_airplane/Vehicle Dynamics/Heading Rate Equation/F_app3/qni ==
  bank1 : Inport
  heading : Inport  Port=2
  latitude : Inport  Port=3
  longitude : Inport  Port=4
  gamma : Inport  Port=5
  get qni : MATLAB Function  TreatAsAtomicUnit=on
  w_earth : Constant  Value=7.2921159e-5
  qni : Outport
  wires:
  bank1/1 -> get qni/1(bank)
  get qni/1(qni) -> qni/1
  latitude/1 -> get qni/5(latitude)
  gamma/1 -> get qni/2(fpa)
  longitude/1 -> get qni/6(longitude)
  heading/1 -> get qni/3(heading)
  w_earth/1 -> get qni/4(we)

== matlab function hf_point_mass_subsonic_airplane/Vehicle Dynamics/Groundspeed Rate Equation/MATLAB Function1 ==
  data: mass input; groundspeed_dot_out output; thrust input; flight_path input; dragOut input; g0 input
function groundspeed_dot_out = fcn(mass, thrust, flight_path, dragOut, g0)
groundspeed_dot_out = (thrust - dragOut)/mass - g0*sind(flight_path);

== matlab function hf_point_mass_subsonic_airplane/Guidance & Control System/Lift Guidance Law & Controller Dynamics/Compute Lift Command/compute sin difference ==
  data: gamma_c input; y output; gamma input
function y = sindifference_fpa(gamma_c, gamma)
y = sind(gamma_c) - sind(gamma);

== matlab function hf_point_mass_subsonic_airplane/Guidance & Control System/Lift Guidance Law & Controller Dynamics/Compute alpha1/2//rho//sw//cla ==
  data: y output; rho input; sw input; cla input
function y = fcn(rho, sw, cla)
y = 2/(rho*sw*cla);

== matlab function hf_point_mass_subsonic_airplane/Guidance & Control System/Lift Guidance Law & Controller Dynamics/Compute alpha/2//rho//sw//cla ==
  data: y output; rho input; sw input; cla input
function y = fcn(rho, sw, cla)
y = 2/(rho*sw*cla);

== matlab function hf_point_mass_subsonic_airplane/Planning System/Command System ==
  data: latitude input; groundspeed_com output; longitude input; altitude input; flight_path_com output; heading_com output
function [groundspeed_com, flight_path_com, heading_com] = ...
    command_trajectory(latitude, longitude, altitude)
% Define the commanded velocity, flight path and heading

FPS2MPH = 3600/5280;
DEG2RAD = pi/180;
RAD2DEG = 180/pi;

groundspeed_com = 450/FPS2MPH;          % fps
flight_path_com = 5*DEG2RAD;    % rad
heading_com = 15*DEG2RAD;          % rad

end

== matlab function hf_point_mass_subsonic_airplane/Vehicle Dynamics/Groundspeed Rate Equation/Fapp_1/MATLAB Function2 ==
  data: longitude input; latitude input; heading input; w_e input; fapp1 output; altitude input; RE input; flight_path input
function fapp1 = fcn(longitude, latitude, heading, w_e, altitude, RE, flight_path)
fapp1 = -w_e.^2 * (RE + altitude) * cosd(latitude) * (sind(latitude)*cosd(flight_path)*cosd(heading) - cosd(latitude)*sind(flight_path));

== matlab function hf_point_mass_subsonic_airplane/Vehicle Dynamics/Groundspeed Rate Equation/High Fidelity Rho/MATLAB Function2 ==
  data: altitude input; ro output
function ro = getRho(altitude)
if altitude < 36089
    ro = 6.6277e-15 * (518.69 - (3.5662e-3)*altitude).^(4.256);
elseif altitude < 65617
    ro = 1.4939e-6 * 2678.4*exp(-4.8063e-5)*altitude;
elseif altitude < 104990
    ro = 2.2099e87*(389.99 + (5.4864e-4)*(altitude-65617)).^(-35.164);
else
    ro = 2.3769e-3;
end

== matlab function hf_point_mass_subsonic_airplane/Vehicle Dynamics/Flight Path Rate Equation/F_app2/rni/get r_ni ==
  data: bank input; rni output; fpa input; heading input; we input; latitude input; longitude input
function rni = getrni(bank,fpa,heading, we, latitude, longitude)
x = [bank, fpa, heading];
C = [cosd(fpa)*cosd(heading) cosd(fpa)*sind(heading) -sind(fpa)
    sind(bank)*sind(fpa)*cosd(heading) - cosd(bank)*sind(heading) sind(bank)*sind(fpa)*sind(heading) + cosd(bank)*cosd(heading) sind(bank)*cosd(fpa)
    cosd(bank)*sind(fpa)*cosd(heading) + sind(bank)*sind(heading) cosd(bank)*sind(fpa)*sind(heading) - sind(bank)*cosd(heading) cosd(bank)*cosd(fpa)];

mat = C*[(we + latitude)*cosd(longitude); -longitude;-(we + latitude)*sind(longitude)];
rni = mat(3);

== matlab function hf_point_mass_subsonic_airplane/Vehicle Dynamics/Flight Path Rate Equation/F_app2/fapp2_term3/MATLAB Function2 ==
  data: longitude input; latitude input; heading input; w_e input; fapp2 output; altitude input; RE input; bank input; flight_path input
function fapp2 = getfapp2term3(longitude, latitude, heading, w_e, altitude, RE, bank, flight_path)
fapp2 = -w_e.^2 * (RE + altitude) * cosd(latitude) * (sind(latitude) * (...
    (sind(bank)*sind(flight_path)*cosd(heading) - cosd(bank)*sind(heading)) + ...
    cosd(latitude)*sind(bank)*cosd(flight_path)));

== matlab function hf_point_mass_subsonic_airplane/Vehicle Dynamics/Flight Path Rate Equation/F_app2/rei/get rei ==
  data: bank input; rei output; fpa input; heading input; we input; latitude input; longitude input
function rei = getrei(bank,fpa,heading, we, latitude, longitude)
x = [bank, fpa, heading];
C = [cosd(fpa)*cosd(heading) cosd(fpa)*sind(heading) -sind(fpa)
    sind(bank)*sind(fpa)*cosd(heading) - cosd(bank)*sind(heading) sind(bank)*sind(fpa)*sind(heading) + cosd(bank)*cosd(heading) sind(bank)*cosd(fpa)
    cosd(bank)*sind(fpa)*cosd(heading) + sind(bank)*sind(heading) cosd(bank)*sind(fpa)*sind(heading) - sind(bank)*cosd(heading) cosd(bank)*cosd(fpa)];

mat = C*[(we)*cosd(longitude); 0;-(we)*sind(longitude)];
rei = mat(3);

== matlab function hf_point_mass_subsonic_airplane/Vehicle Dynamics/Flight Path Rate Equation/F_app3/fapp3_term3/MATLAB Function2 ==
  data: longitude input; latitude input; heading input; w_e input; fapp3 output; altitude input; RE input; bank input; flight_path input
function fapp3 = getFapp3(longitude, latitude, heading, w_e, altitude, RE, bank, flight_path)
fapp3 = -w_e.^2 * (RE + altitude) * cosd(latitude) * (sind(latitude) * (...
    (cosd(bank)*sind(flight_path)*cosd(heading) + sind(bank)*sind(heading)) + ...
    cosd(latitude)*cosd(bank)*cosd(flight_path)));

== matlab function hf_point_mass_subsonic_airplane/Vehicle Dynamics/Flight Path Rate Equation/F_app3/qei/get qei ==
  data: bank input; qei output; fpa input; heading input; we input; latitude input; longitude input
function qei = getqei(bank,fpa,heading, we, latitude, longitude)
x = [bank, fpa, heading];
C = [cosd(fpa)*cosd(heading) cosd(fpa)*sind(heading) -sind(fpa)
    sind(bank)*sind(fpa)*cosd(heading) - cosd(bank)*sind(heading) sind(bank)*sind(fpa)*sind(heading) + cosd(bank)*cosd(heading) sind(bank)*cosd(fpa)
    cosd(bank)*sind(fpa)*cosd(heading) + sind(bank)*sind(heading) cosd(bank)*sind(fpa)*sind(heading) - sind(bank)*cosd(heading) cosd(bank)*cosd(fpa)];

mat = C*[(we)*cosd(longitude); 0;-(we)*sind(longitude)];
qei = mat(2);

== matlab function hf_point_mass_subsonic_airplane/Vehicle Dynamics/Flight Path Rate Equation/F_app3/qni/get qni ==
  data: bank input; qni output; fpa input; heading input; we input; latitude input; longitude input
function qni = getqni(bank,fpa,heading, we, latitude, longitude)
x = [bank, fpa, heading];
C = [cosd(fpa)*cosd(heading) cosd(fpa)*sind(heading) -sind(fpa)
    sind(bank)*sind(fpa)*cosd(heading) - cosd(bank)*sind(heading) sind(bank)*sind(fpa)*sind(heading) + cosd(bank)*cosd(heading) sind(bank)*cosd(fpa)
    cosd(bank)*sind(fpa)*cosd(heading) + sind(bank)*sind(heading) cosd(bank)*sind(fpa)*sind(heading) - sind(bank)*cosd(heading) cosd(bank)*cosd(fpa)];

mat = C*[(we + latitude)*cosd(longitude); -longitude;-(we + latitude)*sind(longitude)];
qni = mat(2);

== matlab function hf_point_mass_subsonic_airplane/Vehicle Dynamics/Heading Rate Equation/F_app2/fapp2_term3/MATLAB Function2 ==
  data: longitude input; latitude input; heading input; w_e input; fapp2 output; altitude input; RE input; bank input; flight_path input
function fapp2 = getfapp2term3(longitude, latitude, heading, w_e, altitude, RE, bank, flight_path)
fapp2 = -w_e.^2 * (RE + altitude) * cosd(latitude) * (sind(latitude) * (...
    (sind(bank)*sind(flight_path)*cosd(heading) - cosd(bank)*sind(heading)) + ...
    cosd(latitude)*sind(bank)*cosd(flight_path)));

== matlab function hf_point_mass_subsonic_airplane/Vehicle Dynamics/Groundspeed Rate Equation/MATLAB Function ==
  data: lift input; dragOut output; airspeed input; rho input; Sw input; cd0 input; AR input; oswald input
function dragOut = getDrag(lift, airspeed, rho, Sw, cd0, AR, oswald)
t1 = 1/2 * rho * Sw * cd0 * airspeed;
t2 = 2/(rho * Sw * pi * AR * oswald);
t3 = lift^2/airspeed;
dragOut = t1 + t2*t3;

== matlab function hf_point_mass_subsonic_airplane/Vehicle Dynamics/Heading Rate Equation/F_app2/rei/get rei ==
  data: bank input; rei output; fpa input; heading input; we input; latitude input; longitude input
function rei = getrei(bank,fpa,heading, we, latitude, longitude)
x = [bank, fpa, heading];
C = [cosd(fpa)*cosd(heading) cosd(fpa)*sind(heading) -sind(fpa)
    sind(bank)*sind(fpa)*cosd(heading) - cosd(bank)*sind(heading) sind(bank)*sind(fpa)*sind(heading) + cosd(bank)*cosd(heading) sind(bank)*cosd(fpa)
    cosd(bank)*sind(fpa)*cosd(heading) + sind(bank)*sind(heading) cosd(bank)*sind(fpa)*sind(heading) - sind(bank)*cosd(heading) cosd(bank)*cosd(fpa)];

mat = C*[(we)*cosd(longitude); 0;-(we)*sind(longitude)];
rei = mat(3);
